simulink model "m_blockrep01"  (Simulink 7.6)
settings: Solver=FixedStepDiscrete  StartTime=0.0  StopTime=10.0  FixedStep=0.1  RelTol=1e-3
PreLoadFcn:
  | TBreak = [-5 -4 -3 -2 -1 0 1 2 3 4 5];
  | TData = [-1 -0.9900 -0.9800 -0.9600 -0.7600 0 0.7600 0.9600 0.9800 0.9900 1];
settings Model: Creator=The MathWorks Inc.  LastModifiedBy=itoy
settings OptimizationCC: ConditionallyExecuteInputs=off  InlineParams=on  InitFltsAndDblsToZero=on  EfficientMapNaN2IntZero=off
settings DebuggingCC: SaveWithParameterizedLinksMsg=none  StrictBusMsg=Warning
settings ConfigComp: Description=Design Verifier Custom Configuration Component  DVBlockReplacement=on  DVBlockReplacementRulesList=sldvdemo_custom_blkrep_rule_sqrt  DVMaxTestCaseSteps=500  DVTestSuiteOptimization=CombinedObjectives

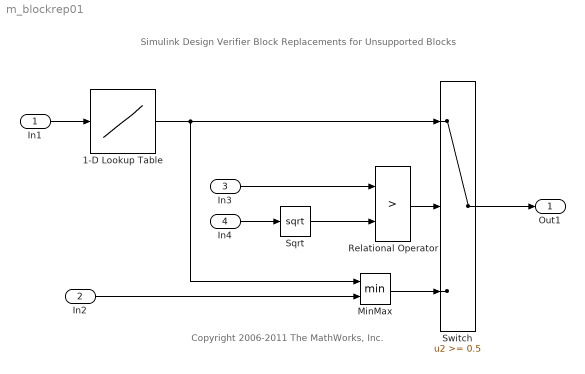
== system m_blockrep01 ==
  note: Simulink Design Verifier
      | Block Replacements for Unsupported Blocks
  note: Copyright 2006-2011 The MathWorks, Inc.
  In1 : Inport
  In2 : Inport  Port=2
  In3 : Inport  Port=3
  In4 : Inport  Port=4
  1-D Lookup Table : Lookup_n-D  NumberOfTableDimensions=1  BreakpointsForDimension1=TData  Table=TBreak  RndMeth=Simplest  InputSameDT=on
  MinMax : MinMax  Inputs=2
  Relational Operator : RelationalOperator  Operator=>  OutDataTypeStr=boolean
  Sqrt : Sqrt  SaturateOnIntegerOverflow=on
  Switch : Switch  Threshold=0.5
  Out1 : Outport
  wires:
  1-D Lookup Table/1 -> Switch/1, MinMax/1
  In2/1 -> MinMax/2
  MinMax/1 -> Switch/3
  In3/1 -> Relational Operator/1
  In4/1 -> Sqrt/1
  Sqrt/1 -> Relational Operator/2
  Relational Operator/1 -> Switch/2
  Switch/1 -> Out1/1
  In1/1 -> 1-D Lookup Table/1
